simulink model "Hbridge"  (R2014a)
settings: Solver=ode23  StartTime=0.0  StopTime=0.01  RelTol=1e-3
libraries: fl_lib x17, elec_lib x16, nesl_utility x6
settings Model: Creator=laca  LastModifiedBy=laca

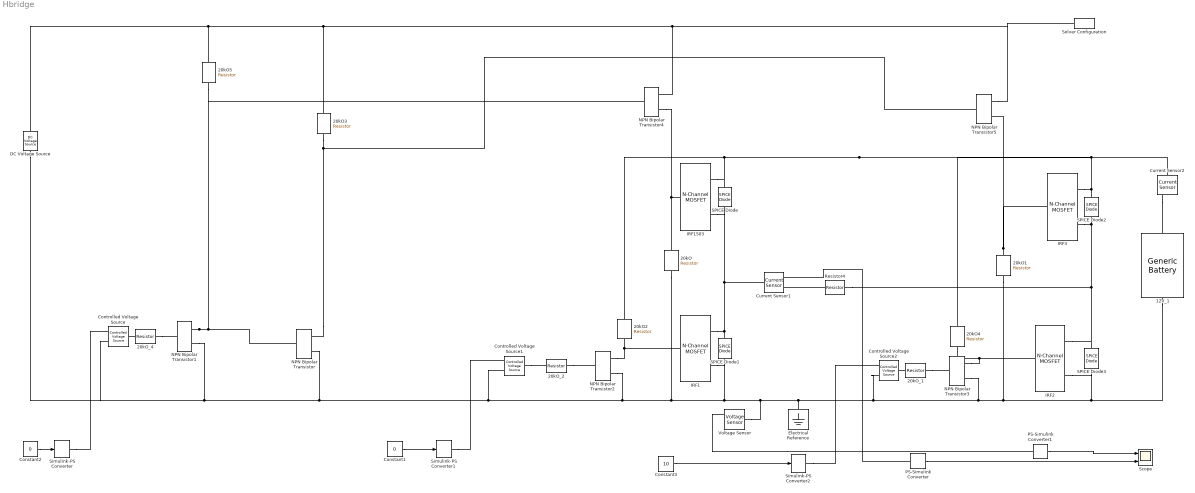
== system Hbridge ==
  12V_1 : elec_lib/Sources/Generic Battery  Vnom=12 V  R1=0.1 Ohm  prm_AH=1  AH=50 hr*A  AH0=50 hr*A  V1=11.5 V  AH1=25 hr*A  prm_R2=1  R2=2e+3 Ohm
  20kO{,1..2,4} (4 alike) : fl_lib/Electrical/Electrical Elements/Resistor  R=20 kOhm  i_specify=off  i_priority=High  i=0 A  v_specify=on  v_priority=High  v=0 V
  20kO3 : fl_lib/Electrical/Electrical Elements/Resistor  R=10 Ohm  i_specify=off  i_priority=High  i=0 A  v_specify=on  v_priority=High  v=0 V
  20kO5 : fl_lib/Electrical/Electrical Elements/Resistor  R=10 Ohm  i_specify=off  i_priority=High  i=0 A  v_specify=on  v_priority=High  v=0 V
  20kO_1 : fl_lib/Electrical/Electrical Elements/Resistor  R=2000 Ohm  i_specify=off  i_priority=High  i=0 A  v_specify=off  v_priority=High  v=0 V
  20kO_2 : fl_lib/Electrical/Electrical Elements/Resistor  R=2000 Ohm  i_specify=off  i_priority=High  i=0 A  v_specify=off  v_priority=High  v=0 V
  20kO_4 : fl_lib/Electrical/Electrical Elements/Resistor  R=20 Ohm  i_specify=off  i_priority=High  i=0 A  v_specify=off  v_priority=High  v=0 V
  Constant1 : Constant  Value=0
  Constant2 : Constant  Value=0
  Constant3 : Constant  Value=10
  Controlled Voltage Source : fl_lib/Electrical/Electrical Sources/Controlled Voltage Source
  Controlled Voltage Source1 : fl_lib/Electrical/Electrical Sources/Controlled Voltage Source
  Controlled Voltage Source2 : fl_lib/Electrical/Electrical Sources/Controlled Voltage Source
  Current Sensor1 : fl_lib/Electrical/Electrical Sensors/Current Sensor
  Current Sensor2 : fl_lib/Electrical/Electrical Sensors/Current Sensor
  DC Voltage Source : elec_lib/Additional Components/SPICE-Compatible Components/Sources/DC Voltage Source  DC=30 V
  Electrical Reference : fl_lib/Electrical/Electrical Elements/Electrical Reference
  IRF{1..3,1503} (4 alike) : elec_lib/Semiconductor Devices/N-Channel MOSFET  parameterization=1  prmDatasheet=1  prmEquCoeff=1  Beta=5 A/V^2  Rds=0.0033 Ohm  Id=75 A  Vgs=10 V  Vth=3 V  lam=0 1/V  Tmeas=25 C  RS=1e-4 Ohm  RD=0.001 Ohm  C_param=1  C_GS=270 pF  C_GD=80 pF  C_iss=5730 pF  C_rss=290 pF  C_oss=2250 pF  charge_linearity_param=1  C_OX=200 pF  V_C_OX=-0.5 V  dVth_dT=-6 mV/K  Rds_T2=0.037 Ohm  Tmeas2=125 C  BEXDatasheet=-1.5  BEXEquCoeff=-1.5  TdeviceDatasheet=25 C  TdeviceEquCoeff=25 C  Rth=[ 0 10 ] K/W  thermal_mass_parameterization=1  thermal_mass=[ 0 1 ] J/K  thermal_time_constant=[ 0 10 ] s  thermal_mass_initial_temperatures=[ 25 25 ] C
  NPN Bipolar Transistor{,1..5} (6 alike) : elec_lib/Semiconductor Devices/NPN Bipolar Transistor  parameterization=1  prmDatasheet=1  prmEquCoeff=1  BF=100  IS=1e-14 A  ec=1  VAF=200 V  hfe=100  hoe=5e-5 1/Ohm  Ic_h=1 mA  Vce_h=5 V  V1=0.55 V  I1=0.5 mA  BR=1  Tmeas=25 C  RC=0.01 Ohm  RE=1e-4 Ohm  RB=1 Ohm  C_BC=5 pF  C_BE=5 pF  TF=0 us  TR=0 us  hfe_T2=125  XTB=0  V1_T2=0.45 V  I1_T2=0.5 mA  Tmeas2=125 C  EG=1.11 eV  XTI=3  TdeviceDatasheet=25 C  TdeviceEquCoeff=25 C  Rth=[ 0 10 ] K/W  thermal_mass_parameterization=1  thermal_mass=[ 0 1 ] J/K  thermal_time_constant=[ 0 10 ] s  thermal_mass_initial_temperatures=[ 25 25 ] C
  PS-Simulink Converter : nesl_utility/PS-Simulink Converter  PhysicalDomain=network_engine_domain  SubClassName=ps_output  LeftPortType=input  RightPortType=output  PseudoPeriodic=off  Frequencies=[]  Unit=1  AffineConversion=off
  PS-Simulink Converter1 : nesl_utility/PS-Simulink Converter  PhysicalDomain=network_engine_domain  SubClassName=ps_output  LeftPortType=input  RightPortType=output  PseudoPeriodic=off  Frequencies=[]  Unit=1  AffineConversion=off
  Resistor4 : fl_lib/Electrical/Electrical Elements/Resistor  R=1 Ohm  i_specify=off  i_priority=High  i=0 A  v_specify=on  v_priority=High  v=0 V
  SPICE Diode{,1..3} (4 alike) : elec_lib/Additional Components/SPICE-Compatible Components/Semiconductor Devices/SPICE Diode  AREA=1 m^2  SCALE=1  IS=1e-14 A/m^2  RS=0.01 m^2*Ohm  ND=1  C_param=1  CJO=0 F/m^2  VJ=1 V  MG=0.5  FC=0.5  TT=0 s  RevBrk=1  BV=Inf V  IBV=0.001 A/m^2  T_param=1  XTI=3  EG=1.11 eV  TOFFSET=0 K  TFIXED=300.15 K  TMEAS=300.15 K  IC_given=1  V0=0 V
  Scope : Scope  NumInputPorts=2
      settings: YMin=-78.5826~-8.92059e-12  YMax=-71.0986~-8.07101e-12
  Simulink-PS Converter : nesl_utility/Simulink-PS Converter  PhysicalDomain=network_engine_domain  SubClassName=ps_input  LeftPortType=input  RightPortType=output  PseudoPeriodic=off  Frequencies=[]  NoiseDistribution=none  NoiseParameters=[]  Unit=1  AffineConversion=off  InputFiltering=off  SimscapeFilterOrder=1  InputFilterTimeConstant=0.001  UdotUserProvided=1
  Simulink-PS Converter1 : nesl_utility/Simulink-PS Converter  PhysicalDomain=network_engine_domain  SubClassName=ps_input  LeftPortType=input  RightPortType=output  PseudoPeriodic=off  Frequencies=[]  NoiseDistribution=none  NoiseParameters=[]  Unit=1  AffineConversion=off  InputFiltering=off  SimscapeFilterOrder=1  InputFilterTimeConstant=0.001  UdotUserProvided=1
  Simulink-PS Converter2 : nesl_utility/Simulink-PS Converter  PhysicalDomain=network_engine_domain  SubClassName=ps_input  LeftPortType=input  RightPortType=output  PseudoPeriodic=off  Frequencies=[]  NoiseDistribution=none  NoiseParameters=[]  Unit=1  AffineConversion=off  InputFiltering=off  SimscapeFilterOrder=1  InputFilterTimeConstant=0.001  UdotUserProvided=1
  Solver Configuration : nesl_utility/Solver Configuration  PhysicalDomain=network_engine_domain  SubClassName=solver  LeftPortType=input  RightPortType=generic  Accelerate=off  Tones=[]  Harmonics=[]  SimulateNoise=off  Profile=off  UseLocalSampling=off  EnableSwitchedLinearOptims=on  FrequencyDomain=off  UseCCode=off  RelTol=0.001  AbsTol=1e-06  MinStep=1e-09  ToWorkspace=off  DoDC=on  ResidualTolerance=1e-3  UseLocalSolver=off  LocalSolverChoice=NE_TRAPEZOIDAL_ADVANCER  LocalSolverSampleTime=.01  DoFixedCost=on  MaxNonlinIter=3  MaxModeIter=2  LinearAlgebra=Sparse  DelaysMemoryBudget=200  AutomaticFiltering=off  FilteringTimeConstant=0.01
  Voltage Sensor : fl_lib/Electrical/Electrical Sensors/Voltage Sensor
  wires:
  PS-Simulink Converter/1 -> Scope/2
  Constant2/1 -> Simulink-PS Converter/1
  Constant1/1 -> Simulink-PS Converter1/1
  Constant3/1 -> Simulink-PS Converter2/1
  PS-Simulink Converter1/1 -> Scope/1
  connections:
  SPICE Diode1/RConn1 -- IRF1503/RConn2 -- SPICE Diode/LConn1 -- Current Sensor1/LConn1 -- IRF1/RConn1
  SPICE Diode2/RConn1 -- 20kO4/LConn1 -- 20kO2/LConn1 -- IRF1503/RConn1 -- SPICE Diode/RConn1 -- Current Sensor2/LConn1 -- IRF3/RConn1
  IRF1503/LConn1 -- NPN Bipolar Transistor4/RConn2 -- 20kO/LConn1
  SPICE Diode2/LConn1 -- SPICE Diode3/RConn1 -- IRF2/RConn1 -- Resistor4/LConn1 -- IRF3/RConn2
  DC Voltage Source/RConn1 -- Controlled Voltage Source/RConn2 -- Controlled Voltage Source1/RConn2 -- NPN Bipolar Transistor2/RConn2 -- 20kO/RConn1 -- Voltage Sensor/LConn1 -- 20kO1/RConn1 -- SPICE Diode3/LConn1 -- IRF2/RConn2 -- 12V_1/RConn1 -- NPN Bipolar Transistor3/RConn2 -- Controlled Voltage Source2/RConn2 -- Electrical Reference/LConn1 -- IRF1/RConn2 -- SPICE Diode1/LConn1 -- NPN Bipolar Transistor/RConn2 -- NPN Bipolar Transistor1/RConn2
  PS-Simulink Converter/LConn1 -- Current Sensor1/RConn1
  20kO1/LConn1 -- NPN Bipolar Transistor5/RConn2 -- IRF3/LConn1
  NPN Bipolar Transistor2/RConn1 -- 20kO2/RConn1 -- IRF1/LConn1
  NPN Bipolar Transistor3/RConn1 -- 20kO4/RConn1 -- IRF2/LConn1
  20kO3/LConn1 -- DC Voltage Source/LConn1 -- 20kO5/LConn1 -- NPN Bipolar Transistor5/RConn1 -- Solver Configuration/RConn1 -- NPN Bipolar Transistor4/RConn1
  20kO3/RConn1 -- NPN Bipolar Transistor/RConn1 -- NPN Bipolar Transistor5/LConn1
  NPN Bipolar Transistor1/RConn1 -- NPN Bipolar Transistor4/LConn1 -- 20kO5/RConn1 -- NPN Bipolar Transistor/LConn1
  20kO_2/RConn1 -- NPN Bipolar Transistor2/LConn1
  Controlled Voltage Source/LConn1 -- 20kO_4/RConn1
  Controlled Voltage Source1/LConn1 -- 20kO_2/LConn1
  20kO_4/LConn1 -- NPN Bipolar Transistor1/LConn1
  Simulink-PS Converter/RConn1 -- Controlled Voltage Source/RConn1
  Resistor4/RConn1 -- Current Sensor1/RConn2
  Simulink-PS Converter1/RConn1 -- Controlled Voltage Source1/RConn1
  Simulink-PS Converter2/RConn1 -- Controlled Voltage Source2/RConn1
  Current Sensor2/RConn2 -- 12V_1/LConn1
  Voltage Sensor/RConn1 -- PS-Simulink Converter1/LConn1
  20kO_1/LConn1 -- Controlled Voltage Source2/LConn1
  20kO_1/RConn1 -- NPN Bipolar Transistor3/LConn1
